simulink model "fromWorkSpace_TestGen18"  (R2017b)
settings: Solver=FixedStepDiscrete  StartTime=0.0  StopTime=10.0  RelTol=1e-3
model workspace (MAT data in the model file):
  X_structure.time = [0; 0.2; 0.4; 0.6; 0.8; 1; 1.2; 1.4; 1.6; 1.8; 2; 2.2; 2.4; 2.6; 2.8; 3; 3.2; 3.4; 3.6; 3.8; 4; 4.2; 4.4; 4.6; 4.8; 5; 5.2; 5.4; 5.6; 5.8; 6; 6.2; 6.4; 6.6; 6.8; 7; 7.2; 7.4; 7.6; 7.8; 8; 8.2; 8.4; 8.6; 8.8; 9; 9.2; 9.4; 9.6; 9.8]
  X_structure.signals.values = [0 0.198669330795 0.389418342309 0.564642473395 0.7173560909 0.841470984808 0.932039085967 0.985449729988 0.999573603042 0.973847630878 0.909297426826 0.80849640382 ... (150 elements, 50x3)]
  X_structure.signals.dimensions = 3
undefined symbols (not defined in the file): Block_TestLib, trigger
settings Model: Creator=ktrinh  LastModifiedBy=ktrinh
settings DebuggingCC: ParameterOverflowMsg=none

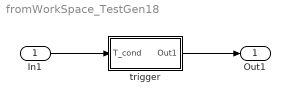
== system fromWorkSpace_TestGen18 ==
  In1 : Inport
  trigger : Subsystem  AncestorBlock=Block_TestLib/trigger
  Out1 : Outport
  wires:
  In1/1 -> trigger/1(T_cond)
  trigger/1(Out1) -> Out1/1

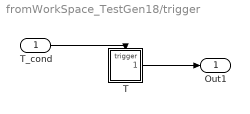
== system fromWorkSpace_TestGen18/trigger ==
  T_cond : Inport  OutDataTypeStr=boolean
  T : Subsystem  TreatAsAtomicUnit=on
  Out1 : Outport
  wires:
  T_cond/1 -> T/Trigger
  T/1(Out1) -> Out1/1

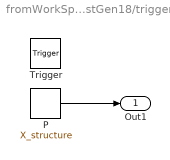
== system fromWorkSpace_TestGen18/trigger/T ==
  Trigger : TriggerPort  VariantControl=Variant
  P : FromWorkspace  VariableName=X_structure  OutputAfterFinalValue=Holding final value
  Out1 : Outport
  wires:
  P/1 -> Out1/1
